simulink model "mod4"  (R2022b)
settings: Solver=VariableStepAuto  StartTime=0.0  StopTime=10.0  RelTol=1e-3
settings Model: Creator=asus  LastModifiedBy=asus

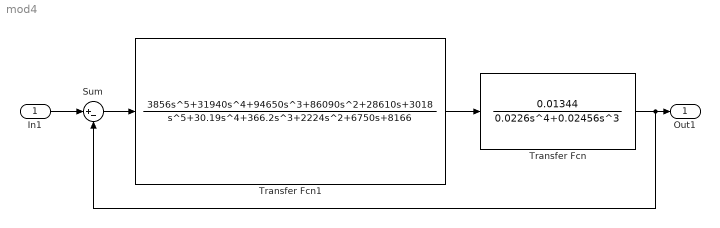
== system mod4 ==
  In1 : Inport
  Sum : Sum  Inputs=|+-
  Transfer Fcn : TransferFcn  Numerator=[0.01344]  Denominator=[0.0226 0.02456 0 0 0]
  Transfer Fcn1 : TransferFcn  Numerator=[3856 31940 94650 86090 28610 3018]  Denominator=[1 30.19 366.2 2224 6750 8166]
  Out1 : Outport
  wires:
  In1/1 -> Sum/1
  Transfer Fcn1/1 -> Transfer Fcn/1
  Transfer Fcn/1 -> Sum/2, Out1/1
  Sum/1 -> Transfer Fcn1/1
